simulink model "mcb_pmsm_host_offsetComputation_f28069m"  (R2024b)
settings: Solver=FixedStepDiscrete  StartTime=0.0  StopTime=inf  RelTol=1e-3  EnableMultiTasking=on
StartFcn:
  | set_param([bdroot '/Serial Communication/Emergency Stop'], 'Value', '1');
undefined symbols (not defined in the file): motor, Ts
libraries: simulink x4, instrumentseriallib x3, mcbcontrolslib x2, mcbpositiondecoderlib x1
settings Model: Creator=The MathWorks, Inc.  LastModifiedBy=The MathWorks, Inc.
settings SolverCC: AlgebraicLoopSolver=TrustRegion  MaxZcPerStep=1
settings DataIOCC: LimitDataPoints=on  SaveFormat=Array  ReturnWorkspaceOutputs=off
settings OptimizationCC: LifeSpan=1  EfficientTunableParamExpr=on
settings DebuggingCC: MergeDetectMultiDrivingBlocksExec=none  SolverPrmCheckMsg=warning  ParameterPrecisionLossMsg=none  UnconnectedInputMsg=warning  UnconnectedOutputMsg=warning  UnconnectedLineMsg=warning  AllowSymbolicDim=off  PregeneratedLibrarySubsystemCodeDiagnostic=none  SFUnexpectedBacktrackingDiag=warning  SFNoUnconditionalDefaultTransitionDiag=warning  SFExecutionAtInitializationDiag=none  ArithmeticOperatorsInVariantConditions=warning
settings HardwareCC: ProdBitPerPointer=32  ProdLargestAtomicFloat=None  ProdIntDivRoundTo=Undefined  ProdEndianess=Unspecified  ProdWordSize=32  ProdHWDeviceType=32-bit Generic
settings ModelReferenceCC: EnableRefExpFcnMdlSchedulingChecks=on  PropagateSignalLabelsOutOfModel=off
settings SFSimCC: SimUseLocalCustomCode=off  MATLABDynamicMemAlloc=off
settings RTWCC: Description=Real-Time Workshop Embedded Coder  SystemTargetFile=ert.tlc  TemplateMakefile=ert_default_tmf  GenerateReport=on  RTWUseLocalCustomCode=off  IncludeHyperlinkInReport=on  LaunchReport=on  GenerateTraceInfo=on  GenerateTraceReport=on  GenerateTraceReportSl=on  GenerateTraceReportSf=on  GenerateTraceReportEml=on  GPUComputeCapability=3.5  DLArmComputeVersion=19.05
settings CodeAppCC: IgnoreCustomStorageClasses=off  StateflowObjectComments=on  InternalIdentifier=Classic
settings ERTTargetCC: MultiwordLength=2048  GenerateSampleERTMain=on  InlinedParameterPlacement=Hierarchical  ERTCustomFileTemplate=example_file_process.tlc  ConvertIfToSwitch=off  SuppressUnreachableDefaultCases=off  DynamicArrayContainerType=coder::array
settings ConfigComp: CovMetricSettings=dw  CovSaveCumulativeToWorkspaceVar=on  CovSaveSingleToWorkspaceVar=on  CovExternalEMLEnable=off  CovSFcnEnable=off

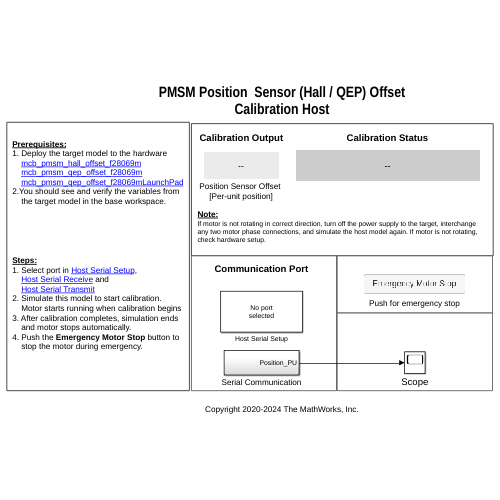
[thumbnail: Simulink's stored preview of the top-level diagram]
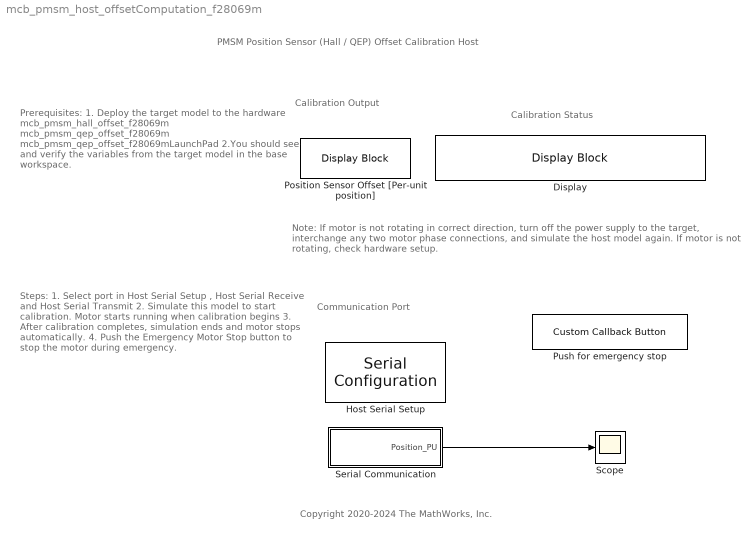
== system mcb_pmsm_host_offsetComputation_f28069m ==
  note: PMSM Position Sensor (Hall / QEP) Offset Calibration Host
  note: Steps:
      | 1. Select port in Host Serial Setup ,
      | Host Serial Receive and
      | Host Serial Transmit
      | 2. Simulate this model to start calibration.
      | Motor starts running when calibration begins
      | 3. After calibration completes, simulation ends
      | and motor stops automatically.
      | 4. Push the Emergency Motor Stop button to
      | stop the motor during emergency.
  note: Prerequisites:
      | 1. Deploy the target model to the hardware
      | mcb_pmsm_hall_offset_f28069m
      | mcb_pmsm_qep_offset_f28069m
      | mcb_pmsm_qep_offset_f28069mLaunchPad
      | 2.You should see and verify the variables from
      | the target model in the base workspace.
  note: Calibration Status
  note: Calibration Output
  note: Communication Port
  note: Copyright 2020-2024 The MathWorks, Inc.
  note: Note:
      | If motor is not rotating in correct direction, turn off the power supply to the target, interchange any two motor phase connections, and simulate the host model again. If motor is not rotating, check hardware setup.
  Display : DisplayBlock  LabelPosition=Hide  Transparency=1
  Host Serial Setup : instrumentseriallib/Serial Configuration  Priority=-99  PortSel=<Select a port...>  Port=<Select a port...>  ComPort=<Select a port...>  BaudRate=5.625e6  DataBits=8  Parity=none  StopBits=1  ByteOrder=little-endian  FlowControl=none  Timeout=2  SimulateUsing=Interpreted execution  BlockInModel=on  aMode=5
      settings: LibrarySourceBlock=mcblib/Protection and Diagnostics/Host Serial Setup
  Position Sensor Offset [Per-unit position] : DisplayBlock  LabelPosition=Hide  Transparency=1
  Push for emergency stop : CustomCallbackButton  Configuration="{\"components\":[{\"name\":\"BackgroundImageComponent\",\"settings\":{\"image\":{\"size\":[0,0],\"src\":\"default\",\"srcOrientation\":\"Right\"},\"position\":[0,0,1,1]}},{\"name\":\"ButtonStateComponent\",\"settings\":{\"buttonType\":\"momentary\",\"clickFcn\":\"set_param([bdroot '\\/Serial Communication\\/Emergency Stop'], 'Value', '0');\",\"onValue\":1,\"position\":[0,0,1,1],\"pressDelay\":\"500\",\"pressFcn\":\"\",\"repeatInterval\":\"0\",\"states\":[{\"horizontalAlignment\":\"center\",\"image\":{\"position\":[0,0,1,1],\"src\":\"default\",\"srcOrientation\":\"Right\"},\"label\":{\"color\":[0.01176470588,0.01176470588,0.01176470588,1],\"icon\":{\"size\":[0,0],\"src\":\"default\",\"srcOrientation\":\"Right\"},\"iconPlacement\":\"left\",\"text\":{\"content\":\"Emergency Motor Stop\"}},\"labelOffset\":[0,0],\"verticalAlignment\":\"middle\"},{\"horizontalAlignment\":\"center\",\"image\":{\"position\":[0,0,1,1],\"src\":\"default\",\"srcOrientation\":\"Right\"},\"label\":{\"color\":[0.01176470588,0.01176470588,0.01176470588,1],\"icon\":{\"size\":[0,0],\"src\":\"default\",\"srcOrientation\":\"Right\"},\"iconPlacement\":\"left\",\"text\":{\"content\":\"Emergency Motor Stop\"}},\"labelOffset\":[0,0],\"verticalAlignment\":\"middle\"},{\"horizontalAlignment\":\"center\",\"image\":{\"position\":[0,0,1,1],\"src\":\"default\",\"srcOrientation\":\"Right\"},\"label\":{\"color\":[0.01176470588,0.01176470588,0.01176470588,1],\"icon\":{\"size\":[0,0],\"src\":\"default\",\"srcOrientation\":\"Right\"},\"iconPlacement\":\"left\",\"text\":{\"content\":\"Emergency Motor Stop\"}},\"labelOffset\":[0,0],\"verticalAlignment\":\"middle\"},{\"horizontalAlignment\":\"center\",\"image\":{\"position\":[0,0,1,1],\"src\":\"default\",\"srcOrientation\":\"Right\"},\"label\":{\"color\":[0.01176470588,0.01176470588,0.01176470588,1],\"icon\":{\"size\":[0,0],\"src\":\"default\",\"srcOrientation\":\"Right\"},\"iconPlacement\":\"left\",\"text\":{\"content\":\"Emergency Motor Stop\"}},\"labelOffset\":[0,0],\"verticalAlignment\":\"middle\"}]}},{\"name\":\"ForegroundImageComponent\",\"settings\":{\"image\":{\"size\":[0,0],\"src\":\"default\",\"srcOrientation\":\"Right\"},\"isForeground\":1,\"position\":[0,0,1,1]}}],\"settings\":{\"BindingType\":\"standalone\",\"backgroundColor\":[244,244,244,1],\"backgroundOffset\":0.2,\"backgroundOpacity\":1,\"fixedAspectRatio\":\"off\",\"foregroundColor\":[0.01176470588,0.01176470588,0.01176470588,1],\"migratedFromLegacy\":true,\"useBackgroundColor\":true,\"variant\":\"callback\",\"version\":\"R2023a\"},\"type\":\"Button\"}"  CustomBackgroundColor="{\"color\":[0.9568627451,0.9568627451,0.9568627451],\"show\":true}"
  Scope : Scope
  Serial Communication : Subsystem
  wires:
  Serial Communication/1(Position_PU) -> Scope/1

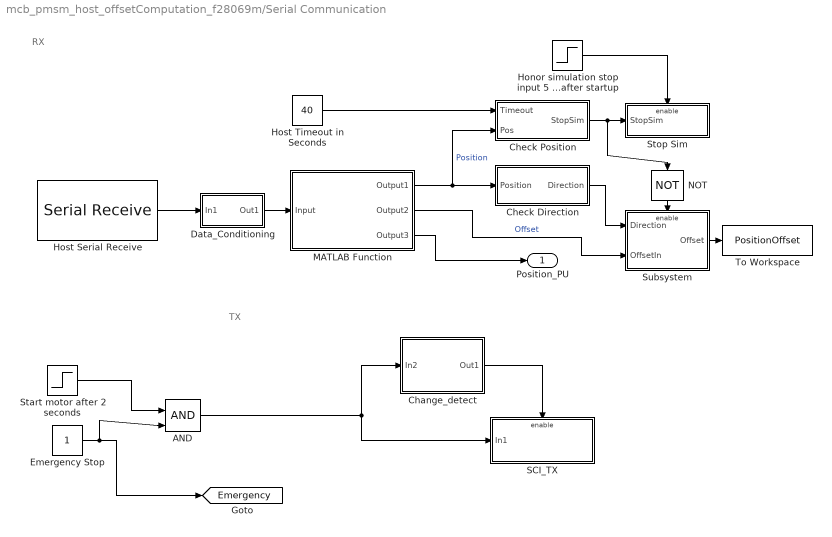
== system mcb_pmsm_host_offsetComputation_f28069m/Serial Communication ==
  note: RX
  note: TX
  AND : Logic  IconShape=distinctive  AllPortsSameDT=off  OutDataTypeStr=boolean
  Change_detect : Subsystem
  Check Direction : Subsystem
  Check Position : Subsystem
  Data_Conditioning : Subsystem
  Emergency Stop : Constant  OutDataTypeStr=Inherit: Inherit via back propagation
  Honor simulation stop input 5 seconds after startup : Step  Time=5  SampleTime=600*Ts
  Host Serial Receive : instrumentseriallib/Serial Receive  PortSel=<Select a port...>  Port=<Select a port...>  ComPort=<Select a port...>  DataType=uint16  SaveDataType=uint8  ToggleHeader=on  Header='SS'  ToggleDataSize=on  DataSize=[600 2]  ToggleTerminator=on  Terminator=Custom terminator  CustomTerminator='EE'  InputFormat=Row major  EnableBlockingMode=on  ActionDataUnavailable=Output custom value  ActionWhenDataUnavailable=Output custom value  CustomValue=4  SampleTime=600*Ts  SimulateUsing=Interpreted execution  BlockInModel=on  aMode=5
      settings: LibrarySourceBlock=mcblib/Protection and Diagnostics/Host Serial Receive
  Host Timeout in Seconds : Constant  Value=40  OutDataTypeStr=Inherit: Inherit via back propagation
  MATLAB Function : MATLAB Function  TreatAsAtomicUnit=on
  NOT : Logic  Operator=NOT  IconShape=distinctive  AllPortsSameDT=off  OutDataTypeStr=boolean
  SCI_TX : Subsystem  TreatAsAtomicUnit=on
  Start motor after 2 seconds : Step  Time=2  OutDataTypeStr=single  SampleTime=Ts*600
  Stop Sim : Subsystem
  Subsystem : Subsystem
  To Workspace : ToWorkspace  VariableName=PositionOffset  SampleTime=-1
      settings: MaxDataPoints=1  Save2DSignal=2-D array (concatenate along first dimension)
  Position_PU : Outport
  tag scope: Emergency=global
  wires:
  MATLAB Function/3(Output3) -> Position_PU/1
  MATLAB Function/2(Output2) -> Subsystem/2(OffsetIn)  "Offset"
  Host Serial Receive/1 -> Data_Conditioning/1(In1)
  MATLAB Function/1(Output1) -> Check Position/2(Pos), Check Direction/1(Position)  "Position"
  Data_Conditioning/1(Out1) -> MATLAB Function/1(Input)
  AND/1 -> SCI_TX/1(In1), Change_detect/1(In2)
  Change_detect/1(Out1) -> SCI_TX/Enable
  Honor simulation stop input 5 seconds after startup/1 -> Stop Sim/Enable
  Check Position/1(StopSim) -> NOT/1, Stop Sim/1(StopSim)
  Check Direction/1(Direction) -> Subsystem/1(Direction)
  NOT/1 -> Subsystem/Enable
  Subsystem/1(Offset) -> To Workspace/1
  Emergency Stop/1 -> [Emergency], AND/2
  Start motor after 2 seconds/1 -> AND/1
  Host Timeout in Seconds/1 -> Check Position/1(Timeout)

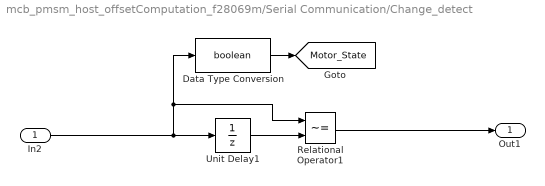
== system mcb_pmsm_host_offsetComputation_f28069m/Serial Communication/Change_detect ==
  In2 : Inport
  Data Type Conversion : DataTypeConversion  OutDataTypeStr=boolean  RndMeth=Simplest  SaturateOnIntegerOverflow=off
  Relational Operator1 : RelationalOperator  Operator=~=  OutDataTypeStr=boolean  InputSameDT=off
  Unit Delay1 : UnitDelay  SampleTime=-1  HasFrameUpgradeWarning=on
  Out1 : Outport  VectorParamsAs1DForOutWhenUnconnected=off
  tag scope: Motor_State=global
  wires:
  In2/1 -> Data Type Conversion/1, Relational Operator1/1, Unit Delay1/1
  Unit Delay1/1 -> Relational Operator1/2
  Relational Operator1/1 -> Out1/1
  Data Type Conversion/1 -> [Motor_State]

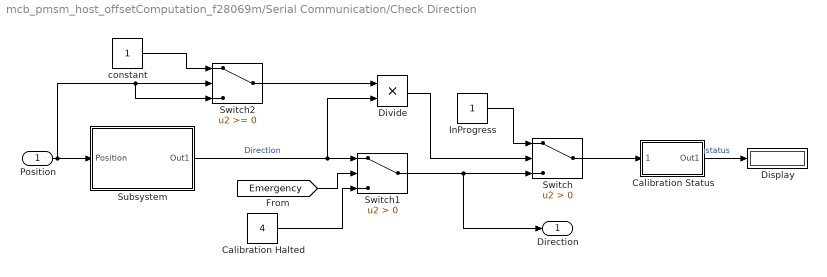
== system mcb_pmsm_host_offsetComputation_f28069m/Serial Communication/Check Direction ==
  Position : Inport
  Calibration Halted : Constant  Value=4  OutDataTypeStr=uint16
  Calibration Status : Subsystem
  Display : Display
  Divide : Product  Inputs=**
  InProgress : Constant  OutDataTypeStr=uint16
  Subsystem : Subsystem
  Switch : Switch  Criteria=u2 > Threshold  SaturateOnIntegerOverflow=off  InputSameDT=off
  Switch1 : Switch  Criteria=u2 > Threshold  SaturateOnIntegerOverflow=off  InputSameDT=off
  Switch2 : Switch  SaturateOnIntegerOverflow=off  InputSameDT=off
  constant : Constant  OutDataTypeStr=uint16
  Direction : Outport
  wires:
  InProgress/1 -> Switch/1
  [Emergency] -> Switch1/2
  Calibration Halted/1 -> Switch1/3
  Switch1/1 -> Direction/1, Switch/3
  Switch/1 -> Calibration Status/1(odataReady)
  Calibration Status/1(Out1) -> Display/1  "status"
  constant/1 -> Switch2/1
  Subsystem/1(Out1) -> Switch1/1, Divide/2  "Direction"
  Switch2/1 -> Divide/1
  Position/1 -> Subsystem/1(Position), Switch2/3, Switch2/2
  Divide/1 -> Switch/2

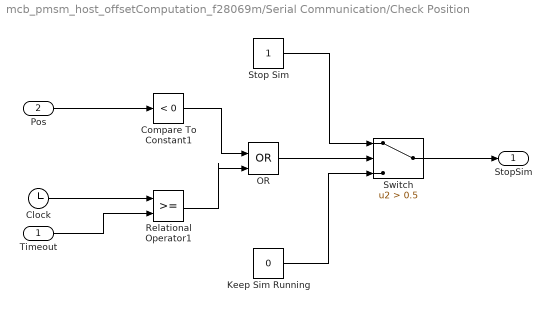
== system mcb_pmsm_host_offsetComputation_f28069m/Serial Communication/Check Position ==
  Timeout : Inport
  Pos : Inport  Port=2
  Clock : Clock
  Compare To Constant1 : simulink/Logic and Bit Operations/Compare To Constant  relop=<  const=0  OutDataTypeStr=boolean
  Keep Sim Running : Constant  Value=0  OutDataTypeStr=Inherit: Inherit via back propagation
  OR : Logic  Operator=OR  IconShape=distinctive  AllPortsSameDT=off  OutDataTypeStr=boolean
  Relational Operator1 : RelationalOperator  OutDataTypeStr=boolean  RndMeth=Simplest  InputSameDT=off
  Stop Sim : Constant  OutDataTypeStr=Inherit: Inherit via back propagation
  Switch : Switch  Criteria=u2 > Threshold  Threshold=0.5  SaturateOnIntegerOverflow=off  InputSameDT=off
  StopSim : Outport
  wires:
  Pos/1 -> Compare To Constant1/1
  Switch/1 -> StopSim/1
  Clock/1 -> Relational Operator1/1
  Compare To Constant1/1 -> OR/1
  Relational Operator1/1 -> OR/2
  OR/1 -> Switch/2
  Stop Sim/1 -> Switch/1
  Keep Sim Running/1 -> Switch/3
  Timeout/1 -> Relational Operator1/2

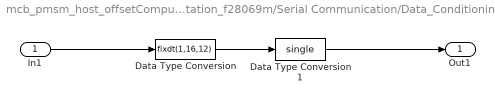
== system mcb_pmsm_host_offsetComputation_f28069m/Serial Communication/Data_Conditioning ==
  In1 : Inport
  Data Type Conversion : DataTypeConversion  OutDataTypeStr=fixdt(1,16,12)  ConvertRealWorld=Stored Integer (SI)  RndMeth=Simplest  SaturateOnIntegerOverflow=off
  Data Type Conversion1 : DataTypeConversion  OutDataTypeStr=single  SaturateOnIntegerOverflow=off  RndMeth=Floor
  Out1 : Outport  VectorParamsAs1DForOutWhenUnconnected=off
  wires:
  Data Type Conversion1/1 -> Out1/1
  In1/1 -> Data Type Conversion/1
  Data Type Conversion/1 -> Data Type Conversion1/1

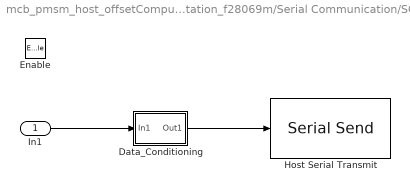
== system mcb_pmsm_host_offsetComputation_f28069m/Serial Communication/SCI_TX ==
  In1 : Inport
  Enable : EnablePort
  Data_Conditioning : Subsystem
  Host Serial Transmit : instrumentseriallib/Serial Send  PortSel=<Select a port...>  Port=<Select a port...>  ComPort=<Select a port...>  Header=[]  Terminator=<none>  CustomTerminator=[]  EnableBlockingMode=off  SimulateUsing=Interpreted execution  BlockInModel=on  aMode=5
      settings: LibrarySourceBlock=mcblib/Protection and Diagnostics/Host Serial Transmit
  wires:
  In1/1 -> Data_Conditioning/1(In1)
  Data_Conditioning/1(Out1) -> Host Serial Transmit/1

== system mcb_pmsm_host_offsetComputation_f28069m/Serial Communication/Stop Sim ==
  StopSim : Inport
  Enable : EnablePort
  Stop Simulation : Stop
  wires:
  StopSim/1 -> Stop Simulation/1

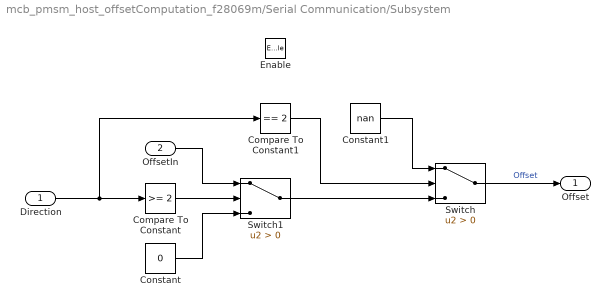
== system mcb_pmsm_host_offsetComputation_f28069m/Serial Communication/Subsystem ==
  Direction : Inport
  OffsetIn : Inport  Port=2
  Enable : EnablePort
  Compare To Constant : simulink/Logic and Bit Operations/Compare To Constant  relop=>=  const=2  OutDataTypeStr=boolean
  Compare To Constant1 : simulink/Logic and Bit Operations/Compare To Constant  relop===  const=2  OutDataTypeStr=boolean
  Constant : Constant  Value=0  OutDataTypeStr=Inherit: Inherit via back propagation
  Constant1 : Constant  Value=nan  OutDataTypeStr=Inherit: Inherit via back propagation
  Switch : Switch  Criteria=u2 > Threshold  SaturateOnIntegerOverflow=off  InputSameDT=off
  Switch1 : Switch  Criteria=u2 > Threshold  SaturateOnIntegerOverflow=off  InputSameDT=off
  Offset : Outport
  wires:
  Switch/1 -> Offset/1  "Offset"
  Direction/1 -> Compare To Constant1/1, Compare To Constant/1
  Constant/1 -> Switch1/3
  Compare To Constant/1 -> Switch1/2
  OffsetIn/1 -> Switch1/1
  Constant1/1 -> Switch/1
  Compare To Constant1/1 -> Switch/2
  Switch1/1 -> Switch/3

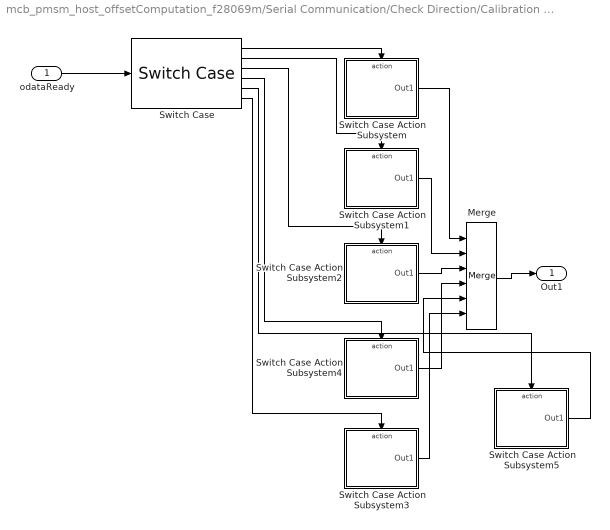
== system mcb_pmsm_host_offsetComputation_f28069m/Serial Communication/Check Direction/Calibration Status ==
  odataReady : Inport
  Merge : Merge  Inputs=6
  Switch Case : SwitchCase  CaseConditions={0,1,2,3,4}
  Switch Case Action Subsystem : Subsystem  TreatAsAtomicUnit=on
  Switch Case Action Subsystem1 : Subsystem  TreatAsAtomicUnit=on
  Switch Case Action Subsystem2 : Subsystem  TreatAsAtomicUnit=on
  Switch Case Action Subsystem3 : Subsystem  TreatAsAtomicUnit=on
  Switch Case Action Subsystem4 : Subsystem  TreatAsAtomicUnit=on
  Switch Case Action Subsystem5 : Subsystem  TreatAsAtomicUnit=on
  Out1 : Outport
  wires:
  Switch Case Action Subsystem4/1(Out1) -> Merge/4
  odataReady/1 -> Switch Case/1
  Switch Case Action Subsystem/1(Out1) -> Merge/1
  Switch Case/4 -> Switch Case Action Subsystem4/Action
  Switch Case/2 -> Switch Case Action Subsystem1/Action
  Switch Case/3 -> Switch Case Action Subsystem2/Action
  Switch Case/1 -> Switch Case Action Subsystem/Action
  Switch Case/6 -> Switch Case Action Subsystem3/Action
  Merge/1 -> Out1/1
  Switch Case Action Subsystem2/1(Out1) -> Merge/3
  Switch Case Action Subsystem1/1(Out1) -> Merge/2
  Switch Case/5 -> Switch Case Action Subsystem5/Action
  Switch Case Action Subsystem3/1(Out1) -> Merge/6
  Switch Case Action Subsystem5/1(Out1) -> Merge/5

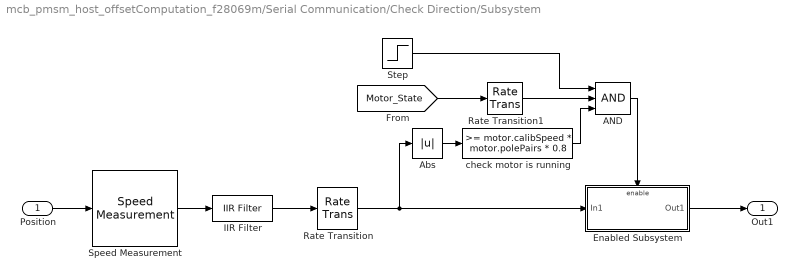
== system mcb_pmsm_host_offsetComputation_f28069m/Serial Communication/Check Direction/Subsystem ==
  Position : Inport
  AND : Logic  Inputs=3  IconShape=distinctive  AllPortsSameDT=off  OutDataTypeStr=boolean
  Abs : Abs  SaturateOnIntegerOverflow=off
  Enabled Subsystem : Subsystem  TreatAsAtomicUnit=on
  IIR Filter : mcbcontrolslib/IIR Filter  VariantControl=Low Pass Filter  VariantSelect=Low-pass  FilterConstantInputType=Specify via dialog  Filter_constant=0.1  advancedSettings=off  Ts=50e-6  cutOff_freq=353.6777
  Rate Transition : RateTransition
  Rate Transition1 : RateTransition
  Speed Measurement : mcbpositiondecoderlib/Speed Measurement  PositionUnit=Per unit  PositionScalingDatatype=uint32  SpeedCalculationMode=Maximum application speed  SampleTimeAsync=Ts*600  MaximumApplicationSpeed=4000  SpeedResolution=5e-6  DelayLength=1  MaximumMeasurableSpeed=0.16484  MeasurableSpeedResolution=7.6757e-11  SpeedUnit=RPM  PerUnitSpeed=1000  SpeedDataType=single
  Step : Step  Time=5  SampleTime=600*Ts
  check motor is running : simulink/Logic and Bit Operations/Compare To Constant  relop=>=  const=motor.calibSpeed * motor.polePairs * 0.8  OutDataTypeStr=boolean
  Out1 : Outport
  wires:
  Rate Transition/1 -> Enabled Subsystem/1(In1), Abs/1
  Rate Transition1/1 -> AND/2
  Abs/1 -> check motor is running/1
  Position/1 -> Speed Measurement/1
  [Motor_State] -> Rate Transition1/1
  check motor is running/1 -> AND/3
  IIR Filter/1 -> Rate Transition/1
  AND/1 -> Enabled Subsystem/Enable
  Speed Measurement/1 -> IIR Filter/1
  Enabled Subsystem/1(Out1) -> Out1/1
  Step/1 -> AND/1

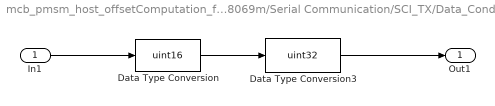
== system mcb_pmsm_host_offsetComputation_f28069m/Serial Communication/SCI_TX/Data_Conditioning ==
  In1 : Inport
  Data Type Conversion : DataTypeConversion  OutDataTypeStr=uint16  RndMeth=Simplest  SaturateOnIntegerOverflow=off
  Data Type Conversion3 : DataTypeConversion  OutDataTypeStr=uint32  ConvertRealWorld=Stored Integer (SI)  RndMeth=Simplest  SaturateOnIntegerOverflow=off
  Out1 : Outport  VectorParamsAs1DForOutWhenUnconnected=off
  wires:
  Data Type Conversion3/1 -> Out1/1
  Data Type Conversion/1 -> Data Type Conversion3/1
  In1/1 -> Data Type Conversion/1

== system mcb_pmsm_host_offsetComputation_f28069m/Serial Communication/Check Direction/Calibration Status/Switch Case Action Subsystem ==
  Action Port : ActionPort
  String Constant : StringConstant  String="\"Motor is not rotating\""
  Out1 : Outport
  wires:
  String Constant/1 -> Out1/1

== system mcb_pmsm_host_offsetComputation_f28069m/Serial Communication/Check Direction/Calibration Status/Switch Case Action Subsystem1 ==
  Action Port : ActionPort
  String Constant : StringConstant  String="\"Calibration is in-progress\""
  Out1 : Outport
  wires:
  String Constant/1 -> Out1/1

== system mcb_pmsm_host_offsetComputation_f28069m/Serial Communication/Check Direction/Calibration Status/Switch Case Action Subsystem2 ==
  Action Port : ActionPort
  String Constant : StringConstant  String="\"Motor not rotating in correct direction\""
  Out1 : Outport
  wires:
  String Constant/1 -> Out1/1

== system mcb_pmsm_host_offsetComputation_f28069m/Serial Communication/Check Direction/Calibration Status/Switch Case Action Subsystem3 ==
  Action Port : ActionPort
  String Constant : StringConstant  String="\"\""
  Out1 : Outport
  wires:
  String Constant/1 -> Out1/1

== system mcb_pmsm_host_offsetComputation_f28069m/Serial Communication/Check Direction/Calibration Status/Switch Case Action Subsystem4 ==
  Action Port : ActionPort
  String Constant : StringConstant  String="\"Calibration Success\""
  Out1 : Outport
  wires:
  String Constant/1 -> Out1/1

== system mcb_pmsm_host_offsetComputation_f28069m/Serial Communication/Check Direction/Calibration Status/Switch Case Action Subsystem5 ==
  Action Port : ActionPort  ActionPortLabel=case [ 4 ]:
  String Constant : StringConstant  String="\"Calibration Halted\""
  Out1 : Outport
  wires:
  String Constant/1 -> Out1/1

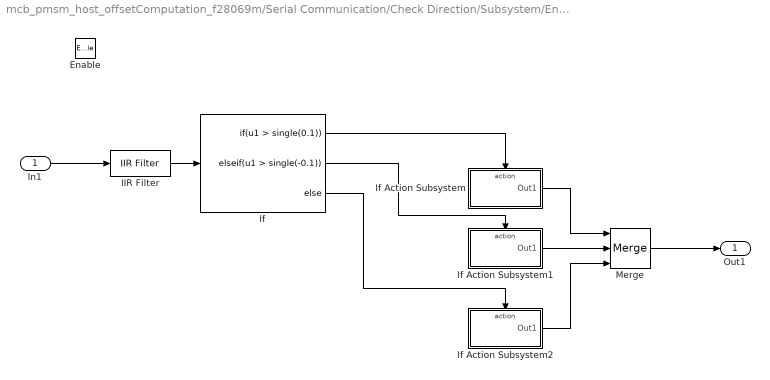
== system mcb_pmsm_host_offsetComputation_f28069m/Serial Communication/Check Direction/Subsystem/Enabled Subsystem ==
  In1 : Inport
  Enable : EnablePort
  IIR Filter : mcbcontrolslib/IIR Filter  VariantControl=Low Pass Filter  VariantSelect=Low-pass  FilterConstantInputType=Specify via dialog  Filter_constant=0.001  advancedSettings=off  Ts=50e-6  cutOff_freq=3.1863
  If : If  IfExpression=u1 > single(0.1)  ElseIfExpressions=u1 > single(-0.1)
  If Action Subsystem : Subsystem  TreatAsAtomicUnit=on
  If Action Subsystem1 : Subsystem  TreatAsAtomicUnit=on
  If Action Subsystem2 : Subsystem  TreatAsAtomicUnit=on
  Merge : Merge  Inputs=3
  Out1 : Outport
  wires:
  In1/1 -> IIR Filter/1
  If/1 -> If Action Subsystem/Action
  If/2 -> If Action Subsystem1/Action
  If/3 -> If Action Subsystem2/Action
  If Action Subsystem/1(Out1) -> Merge/1
  If Action Subsystem1/1(Out1) -> Merge/2
  If Action Subsystem2/1(Out1) -> Merge/3
  IIR Filter/1 -> If/1
  Merge/1 -> Out1/1

== system mcb_pmsm_host_offsetComputation_f28069m/Serial Communication/Check Direction/Subsystem/Enabled Subsystem/If Action Subsystem ==
  Action Port : ActionPort  ActionPortLabel=if(u1 > single(0.1))
  Motor rotating in correct direction : Constant  Value=3  OutDataTypeStr=uint16
  Out1 : Outport
  wires:
  Motor rotating in correct direction/1 -> Out1/1

== system mcb_pmsm_host_offsetComputation_f28069m/Serial Communication/Check Direction/Subsystem/Enabled Subsystem/If Action Subsystem1 ==
  Action Port : ActionPort  ActionPortLabel=elseif(u1 > single(-0.1))
  Motor not rotating : Constant  Value=0  OutDataTypeStr=uint16
  Out1 : Outport
  wires:
  Motor not rotating/1 -> Out1/1

== system mcb_pmsm_host_offsetComputation_f28069m/Serial Communication/Check Direction/Subsystem/Enabled Subsystem/If Action Subsystem2 ==
  Action Port : ActionPort  ActionPortLabel=else
  Motor rotating in wrong direction : Constant  Value=2  OutDataTypeStr=uint16
  Out1 : Outport
  wires:
  Motor rotating in wrong direction/1 -> Out1/1

== matlab function mcb_pmsm_host_offsetComputation_f28069m/Serial Communication/MATLAB Function ==
  data: Output1 output; Output2 output; Output3 output; Input input
function [Output1, Output2, Output3] = unBuf(Input)

selSignal= Input(:, 1);
Output1 = selSignal(1,1);
selSignal = Input(:, 2);
Output2 = selSignal(1,1);
Output3 = Input(:,1);
end
